simulink model "dynamic_systems_everyone"  (R2022b)
settings: Solver=VariableStepAuto  StartTime=0.0  StopTime=10.0  RelTol=1e-3
undefined symbols (not defined in the file): A1, v1, v2
settings Model: Creator=anton  LastModifiedBy=anton

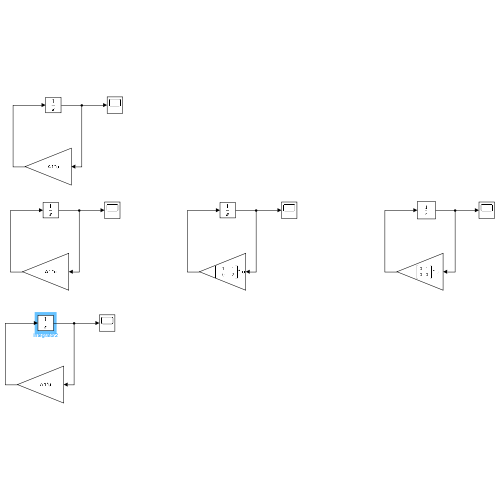
[thumbnail: Simulink's stored preview of the top-level diagram]
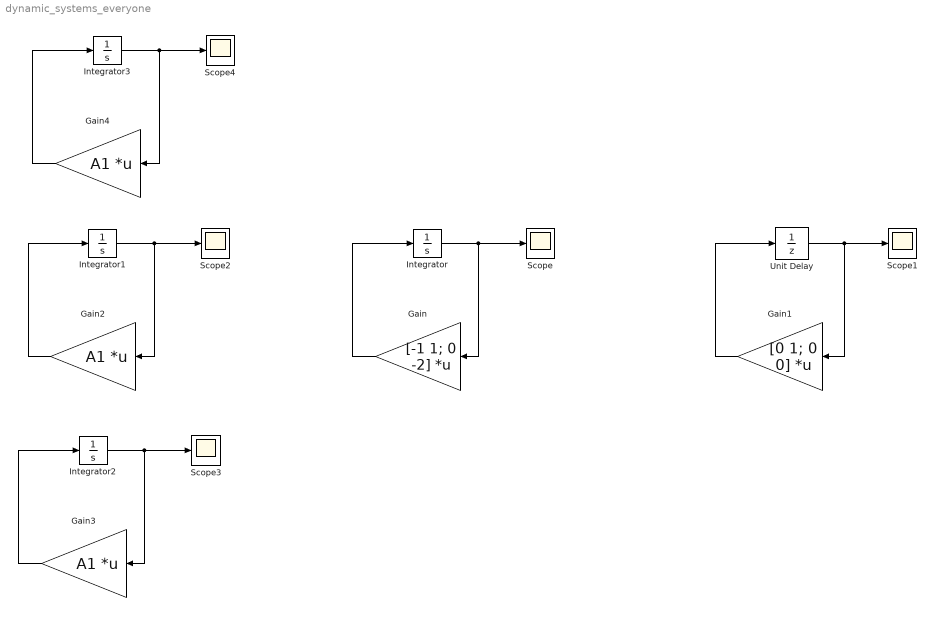
== system dynamic_systems_everyone ==
  Gain : Gain  Gain=[-1 1; 0 -2]  Multiplication=Matrix(K*u)
  Gain1 : Gain  Gain=[0 1; 0 0]  Multiplication=Matrix(K*u)
  Gain2 : Gain  Gain=A1  Multiplication=Matrix(K*u)
  Gain3 : Gain  Gain=A1  Multiplication=Matrix(K*u)
  Gain4 : Gain  Gain=A1  Multiplication=Matrix(K*u)
  Integrator : Integrator  InitialCondition=[2; 3]
  Integrator1 : Integrator  InitialCondition=v2
  Integrator2 : Integrator  InitialCondition=v1
  Integrator3 : Integrator  InitialCondition=[10;-5]
  Scope{,1..4} (5 alike) : Scope
  Unit Delay : UnitDelay  InitialCondition=[2;10]  SampleTime=-1  HasFrameUpgradeWarning=on
  wires:
  Gain/1 -> Integrator/1
  Integrator/1 -> Gain/1, Scope/1
  Gain1/1 -> Unit Delay/1
  Unit Delay/1 -> Gain1/1, Scope1/1
  Integrator1/1 -> Gain2/1, Scope2/1
  Gain2/1 -> Integrator1/1
  Gain3/1 -> Integrator2/1
  Integrator2/1 -> Gain3/1, Scope3/1
  Integrator3/1 -> Gain4/1, Scope4/1
  Gain4/1 -> Integrator3/1
